simulink model "study"  (R2022b)
settings: Solver=ode45  StartTime=0.0  StopTime=60  RelTol=1e-3  EnableMultiTasking=on
undefined symbols (not defined in the file or in its folder): clock
libraries: rllib x1, simulink x1, simulink_extras x1
settings Model: Creator=The MathWorks, Inc.  LastModifiedBy=beikuzi
settings SolverCC: AlgebraicLoopSolver=TrustRegion
settings DataIOCC: LimitDataPoints=on  SaveFormat=Array  ReturnWorkspaceOutputs=off  SignalLoggingName=logsOut
settings OptimizationCC: ExpressionDepthLimit=2147483647  InitFltsAndDblsToZero=on  LifeSpan=inf
settings DebuggingCC: SaveWithParameterizedLinksMsg=none  UnderspecifiedInitializationDetection=Classic  MergeDetectMultiDrivingBlocksExec=none  SignalResolutionControl=TryResolveAllWithWarning  MultiTaskDSMMsg=warning  FcnCallInpInsideContextMsg=warning  UnconnectedInputMsg=warning  UnconnectedOutputMsg=warning  UnconnectedLineMsg=warning  AllowSymbolicDim=off  StateNameClashWarn=warning  SFUnexpectedBacktrackingDiag=warning  SFNoUnconditionalDefaultTransitionDiag=warning  SFExecutionAtInitializationDiag=none  SFMachineParentedDataDiag=warning  ArithmeticOperatorsInVariantConditions=warning
settings HardwareCC: ProdBitPerPointer=32  ProdBitPerSizeT=32  ProdBitPerPtrDiffT=32  ProdLargestAtomicFloat=None  ProdIntDivRoundTo=Undefined  ProdEndianess=Unspecified  ProdWordSize=32  ProdHWDeviceType=Specified
settings ModelReferenceCC: EnableRefExpFcnMdlSchedulingChecks=on  PropagateSignalLabelsOutOfModel=off
settings SFSimCC: SimUseLocalCustomCode=off
settings RTWCC: RTWUseLocalCustomCode=off
settings CodeAppCC: StateflowObjectComments=on
settings GRTTargetCC: TargetFcnLib=ansi_tfl_tmw.mat  TargetLangStandard=C89/C90 (ANSI)  CombineOutputUpdateFcns=off  GRTInterface=on
settings ConfigComp: CovMetricSettings=dw  CovSaveCumulativeToWorkspaceVar=on  CovSaveSingleToWorkspaceVar=on  CovExternalEMLEnable=off

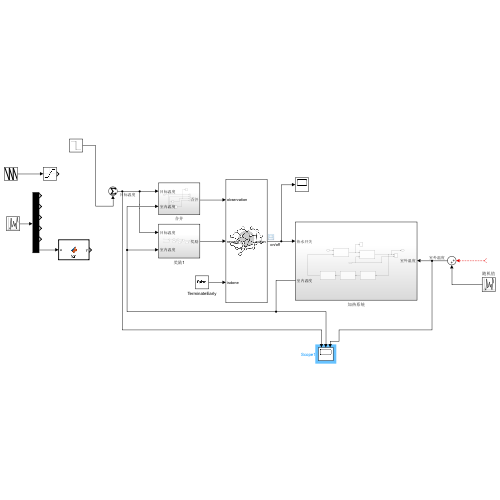
[thumbnail: Simulink's stored preview of the top-level diagram]
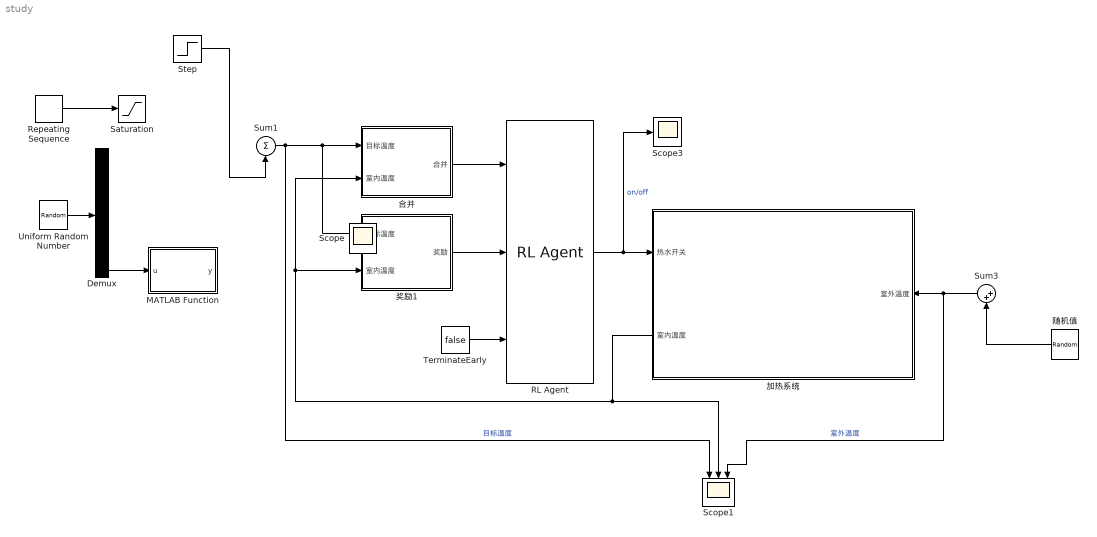
== system study ==
  Demux : Demux  Outputs=6
  MATLAB Function : MATLAB Function  TreatAsAtomicUnit=on
  RL Agent : rllib/RL Agent  Agent=myAgent  ExternalActionAsInput=off  ProvideLastAction=off  ProvideCumRwd=off  TreatAsDirectFeedthrough=on  UseStrictObservationDataTypes=off
  Repeating Sequence : simulink/Sources/Repeating Sequence  rep_seq_t=[0 61]  rep_seq_y=[120 -2]
  Saturation : Saturate  UpperLimit=90  LowerLimit=30
  Scope1 : Scope  NumInputPorts=3
  Scope3 : Scope
  Step : Step  Time=2  Before=50  After=30  SampleTime=0
  Sum1 : Sum  Inputs=|+  InputSameDT=on  SaturateOnIntegerOverflow=on  OutDataTypeStr=Inherit: Same as first input
  Sum3 : Sum  Inputs=|++  InputSameDT=on  SaturateOnIntegerOverflow=on  OutDataTypeStr=Inherit: Same as first input
  TerminateEarly : Constant  Value=false
  Uniform Random Number : UniformRandomNumber  Minimum=0  Seed=round(clock)*1000+randi([1,100])  SampleTime=0.1
  加热系统 : Subsystem
      settings: PortSchema="{\"entries\":[{\"content\":{\"sides\":[{\"content\":{\"connectorIds\":[\"In1\",\"Out1\"]},\"type\":\"ConnectorPlacement.EquallySpacedRectSide\",\"uuid\":\"9f70e1aa-b3a0-450d-b561-7dbc5ba70b42\"},{\"content\":{\"connectorIds\":[\"In2\"],\"side\":\"RIGHT\"},\"type\":\"ConnectorPlacement.EquallySpacedRectSide\",\"uuid\":\"8b3166b5-bb13-401f-8a8b-5c7ef3964e66\"},{\"content\":{\"connectorIds\":[],\"side\":\"TOP\"},\"type\":\"ConnectorPlacement.EquallySpacedRectSide\",\"uuid\":\"6fdb77f1-414f-45ef-bf08-fec8cca9e6c1\"}]},\"type\":\"ConnectorPlacement.EquallySpacedConnector\",\"uuid\":\"8628a7d7-6e87-4572-9342-fd852d46d2e3\"}],\"packageUris\":[\"http://schema.mathworks.com/mf0/Connector/R2020b\"],\"version\":\"1.0\"}"
  合并 : Subsystem
  奖励1 : Subsystem
  随机值 : UniformRandomNumber  Minimum=5  Maximum=20  SampleTime=0.01
  Scope : Scope
  wires:
  RL Agent/1 -> Scope3/1, 加热系统/1(热水开关)  "on/off"
  合并/1(合并) -> RL Agent/1
  ? -> Sum3/1
  Sum3/1 -> Scope1/3, 加热系统/2(室外温度)  "室外温度"
  随机值/1 -> Sum3/2
  加热系统/1(室内温度) -> Scope1/2, 奖励1/2(室内温度), 合并/2(室内温度)
  TerminateEarly/1 -> RL Agent/3
  奖励1/1(奖励) -> RL Agent/2
  Uniform Random Number/1 -> Demux/1
  Demux/6 -> MATLAB Function/1(u)
  Sum1/1 -> Scope1/1, 奖励1/1(目标温度), 合并/1(目标温度)  "目标温度"
  Repeating Sequence/1 -> Saturation/1
  Step/1 -> Sum1/1

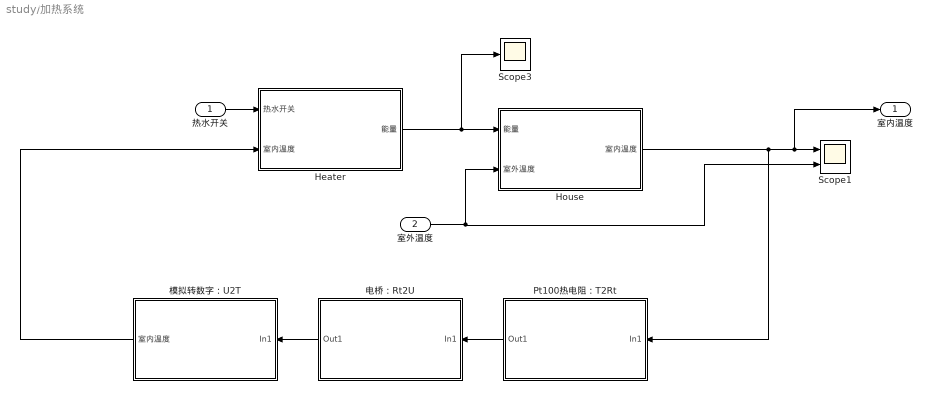
== system study/加热系统 ==
  热水开关 : Inport  OutMin=[0]  OutMax=[1]
  室外温度 : Inport  Port=2  OutMin=[0]  OutMax=[1]
  Heater : Subsystem
  House : Subsystem
  Pt100热电阻：T2Rt : Subsystem
  Scope1 : Scope  NumInputPorts=2
  Scope3 : Scope
  模拟转数字：U2T : Subsystem
  电桥：Rt2U : Subsystem
  室内温度 : Outport
  wires:
  Pt100热电阻：T2Rt/1(Out1) -> 电桥：Rt2U/1(In1)
  Heater/1(能量) -> Scope3/1, House/1(能量)
  热水开关/1 -> Heater/1(热水开关)
  电桥：Rt2U/1(Out1) -> 模拟转数字：U2T/1(In1)
  室外温度/1 -> House/2(室外温度), Scope1/2
  模拟转数字：U2T/1(室内温度) -> Heater/2(室内温度)
  House/1(室内温度) -> 室内温度/1, Scope1/1, Pt100热电阻：T2Rt/1(In1)

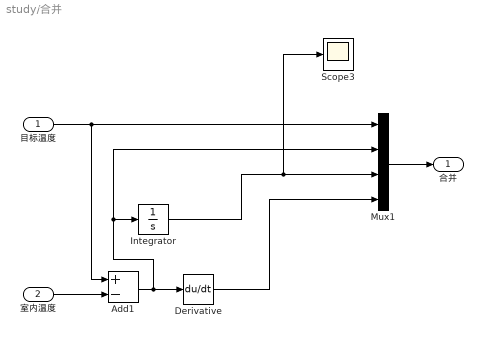
== system study/合并 ==
  目标温度 : Inport  OutMin=[0]  OutMax=[1]
  室内温度 : Inport  Port=2  OutMin=[0]  OutMax=[1]
  Add1 : Sum  Inputs=+-
  Derivative : Derivative
  Integrator : Integrator
  Mux1 : Mux
  Scope3 : Scope
  合并 : Outport
  wires:
  Mux1/1 -> 合并/1
  室内温度/1 -> Add1/2
  目标温度/1 -> Mux1/1, Add1/1
  Add1/1 -> Mux1/2, Integrator/1, Derivative/1
  Derivative/1 -> Mux1/4
  Integrator/1 -> Scope3/1, Mux1/3

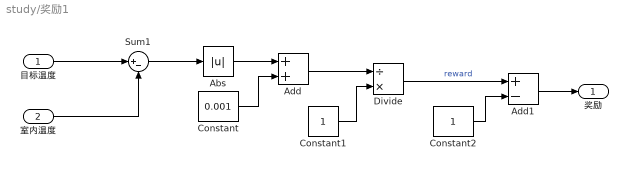
== system study/奖励1 ==
  目标温度 : Inport  OutMin=[0]  OutMax=[1]
  室内温度 : Inport  Port=2  OutMin=[0]  OutMax=[1]
  Abs : Abs  SaturateOnIntegerOverflow=off
  Add : Sum
  Add1 : Sum  Inputs=+-
  Constant : Constant  Value=0.001
  Constant1 : Constant
  Constant2 : Constant
  Divide : Product  Inputs=/*
  Sum1 : Sum  Inputs=|+-  SaturateOnIntegerOverflow=on
  奖励 : Outport
  wires:
  Constant1/1 -> Divide/2
  Constant/1 -> Add/2
  Add/1 -> Divide/1
  Abs/1 -> Add/1
  目标温度/1 -> Sum1/1
  室内温度/1 -> Sum1/2
  Sum1/1 -> Abs/1
  Constant2/1 -> Add1/2
  Divide/1 -> Add1/1  "reward"
  Add1/1 -> 奖励/1

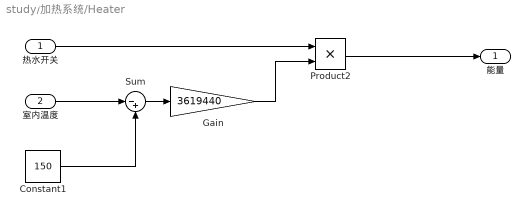
== system study/加热系统/Heater ==
  热水开关 : Inport  OutMin=[0]  OutMax=[1]
  室内温度 : Inport  Port=2
  Constant1 : Constant  Value=150
  Gain : Gain  Gain=3619440
  Product2 : Product
  Sum : Sum  Inputs=|-+
  能量 : Outport
  wires:
  室内温度/1 -> Sum/1
  Constant1/1 -> Sum/2
  Sum/1 -> Gain/1
  热水开关/1 -> Product2/1
  Gain/1 -> Product2/2
  Product2/1 -> 能量/1

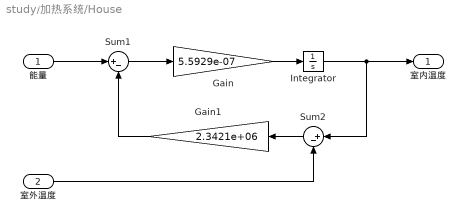
== system study/加热系统/House ==
  能量 : Inport  OutMin=[0]  OutMax=[1]
  室外温度 : Inport  Port=2
  Gain : Gain  Gain=5.5929e-07
  Gain1 : Gain  Gain=2.3421e+06
  Integrator : Integrator  InitialCondition=20
  Sum1 : Sum  Inputs=|+-
  Sum2 : Sum  Inputs=|+-
  室内温度 : Outport
  wires:
  室外温度/1 -> Sum2/2
  能量/1 -> Sum1/1
  Sum1/1 -> Gain/1
  Sum2/1 -> Gain1/1
  Gain1/1 -> Sum1/2
  Gain/1 -> Integrator/1
  Integrator/1 -> Sum2/1, 室内温度/1

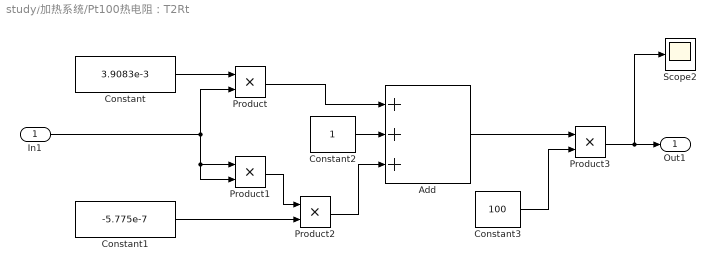
== system study/加热系统/Pt100热电阻：T2Rt ==
  In1 : Inport
  Add : Sum  Inputs=+++
  Constant : Constant  Value=3.9083e-3
  Constant1 : Constant  Value=-5.775e-7
  Constant2 : Constant
  Constant3 : Constant  Value=100
  Product{,1..3} (4 alike) : Product
  Scope2 : Scope
  Out1 : Outport
  wires:
  In1/1 -> Product/2, Product1/2, Product1/1
  Constant/1 -> Product/1
  Constant1/1 -> Product2/2
  Product1/1 -> Product2/1
  Product/1 -> Add/1
  Product2/1 -> Add/3
  Constant2/1 -> Add/2
  Product3/1 -> Scope2/1, Out1/1
  Add/1 -> Product3/1
  Constant3/1 -> Product3/2

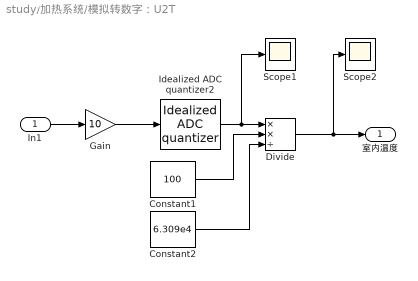
== system study/加热系统/模拟转数字：U2T ==
  In1 : Inport
  Constant1 : Constant  Value=100
  Constant2 : Constant  Value=6.309e4
  Divide : Product  Inputs=**/
  Gain : Gain  Gain=10
  Idealized ADC quantizer2 : simulink_extras/Additional Discrete/Idealized ADC quantizer  NumberOfConverterBits=16  Vmin=0  Vmax=5  OutputDataType=int32  OutputNegativeValues=off
  Scope1 : Scope
  Scope2 : Scope
  室内温度 : Outport
  wires:
  Idealized ADC quantizer2/1 -> Scope1/1, Divide/1
  Constant1/1 -> Divide/2
  Constant2/1 -> Divide/3
  Divide/1 -> Scope2/1, 室内温度/1
  In1/1 -> Gain/1
  Gain/1 -> Idealized ADC quantizer2/1

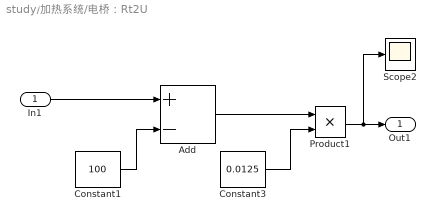
== system study/加热系统/电桥：Rt2U ==
  In1 : Inport
  Add : Sum  Inputs=+-
  Constant1 : Constant  Value=100
  Constant3 : Constant  Value=0.0125
  Product1 : Product
  Scope2 : Scope
  Out1 : Outport
  wires:
  In1/1 -> Add/1
  Constant1/1 -> Add/2
  Add/1 -> Product1/1
  Constant3/1 -> Product1/2
  Product1/1 -> Scope2/1, Out1/1

== matlab function study/MATLAB Function ==
  data: y output; u input
function y = fcn(u)
persistent T;
if isempty(T)  % 检查持久变量是否为空
    T=70*u+20;
    disp(T);
end
y = T;
